simulink model "forward_facing_model"  (R2024b)
settings: Solver=VariableStepAuto  StartTime=0.0  StopTime=2474  RelTol=1e-3
model workspace (MATLAB code in the model file):
  | x = linspace(0,230.4,100);
  | m = 280;
libraries: autolibshared x2
settings Model: Creator=asus  LastModifiedBy=asus

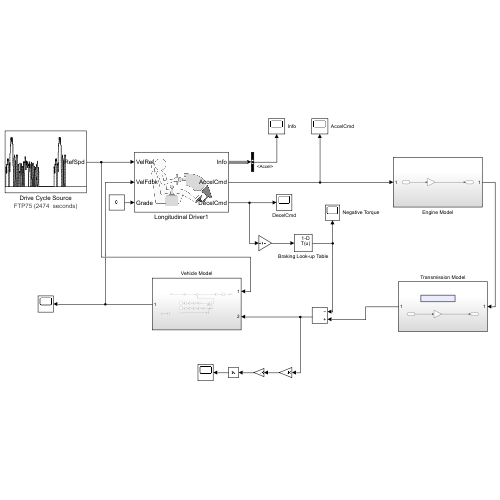
[thumbnail: Simulink's stored preview of the top-level diagram]
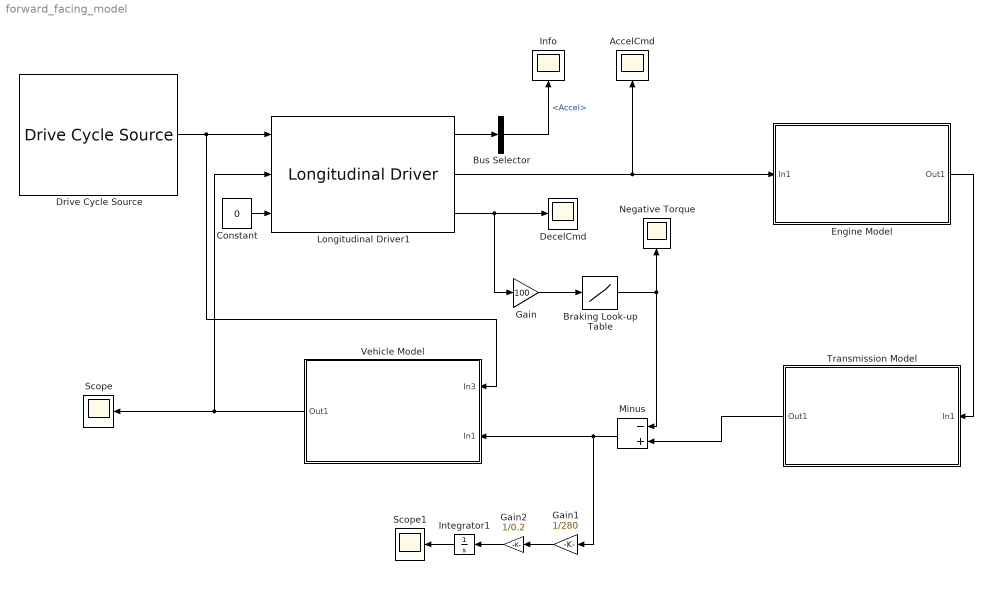
== system forward_facing_model ==
  AccelCmd : Scope
  Braking Look-up Table : Lookup_n-D  NumberOfTableDimensions=1  BreakpointsForDimension1=1:100  Table=x  InternalRulePriority=Speed  RndMeth=Simplest
  Bus Selector : BusSelector  OutputSignals=Accel
  Constant : Constant  Value=0
  DecelCmd : Scope
  Drive Cycle Source : autolibshared/Drive Cycle Source  cycleVar=FTP75  fileVar=cycleFTP75.mat  tfinal="2474  seconds"  cycleRepeat=off  outAccPort=off  outGearPort=off  gearList=No gear data  t_wot1=5  xdot_woto=0  xdot_wot1=30  t_wot2=20  xdot_wot2=0  t_wotend=30  srcUnit=m/s  outUnit=m/s  srcAccUnit=m/s/s  outAccUnit=m/s^2  dt=0  aMode=1  faultOption=off  velBnd=2  velBndUnit=mph  inUnit=m/s  timeBnd=1  failOption=off  stopSim=off  maxFaultCnt=10  maxFaultTime=2  maxTotFaultTime=15  traceOption=off  dtTrace=1  traceWindow=10  lastDCname=FTP75  lastOutUnit=mph  lastDT=0  lastTB=1  lastSB=2  forceCalcBound=off
  Engine Model : Subsystem
  Gain : Gain  Gain=100
  Gain1 : Gain  Gain=1/280
  Gain2 : Gain  Gain=1/0.2
  Info : Scope
  Integrator1 : Integrator
  Longitudinal Driver1 : autolibshared/Longitudinal Driver  extAccelOvr=off  extDecelOvr=off  extAccelHld=off  extDecelHld=off  extAccelZero=off  extDecelZero=off  cntrlType=PI  shftType=None  velUnits=m/s  gearOut=off  Kp=10  Ki=5  Kff=.1  Kg=0  VehVelVec=[0 100]  KffVec=[.1 .1]  KpVec=[10 10]  KiVec=[5 5]  KgVec=[0 0]  m=1500  Kpt=3000  tau=.1  L=2  aR=200  bR=2.5  cR=.5  g=9.81  vnom=5  Kaw=1  tauerr=.01  tauPt=2  GearInit=0  tShift=.1  pdlVec=[0.1 0.4 0.5 0.9]  upShftTbl=[-1 12.9375 26.4375 39.9375 51.18749999999999 62.4375 72.84375 83.25;-1 16.3125 29.8125 43.3125 54.5624 65.8125 76.78125 87.75;-1 19.6875 33.1875 46.68749999999999 57.9375 69.1875 80.71875 92.25;-1 33 52.5 77.25 100.5 138.75 161.875 185]  dwnShftTbl=[1 9.5625 23.0625 36.5625 47.8125 59.0625 68.90625 78.75;1 12.9375 26.4375 39.9375 51.18749999999999 62.4375 72.84375 83.25;1 16.3125 29.8125 43.3125 54.562499 65.8125 76.78125 87.75;1 19.6875 33.1875 46.68749999999999 57.9375 69.1875 80.71875 92.25]  tClutch=.5  tRev=.5  tPark=120  aMode=2  UpGearVec="[0  1  2  3  4  5  6  7]"  DownGearVec="[1  2  3  4  5  6  7  8]"
      settings: LibrarySourceBlock=vehdynlibdriver/Longitudinal Driver
  Minus : Sum  Inputs=-+
  Negative Torque : Scope
  Scope : Scope
  Scope1 : Scope
  Transmission Model : Subsystem
  Vehicle Model : Subsystem
  wires:
  Drive Cycle Source/1 -> Vehicle Model/1(In3), Longitudinal Driver1/1
  Longitudinal Driver1/1 -> Bus Selector/1
  Constant/1 -> Longitudinal Driver1/3
  Bus Selector/1 -> Info/1  "<Accel>"
  Longitudinal Driver1/2 -> Engine Model/1(In1), AccelCmd/1
  Longitudinal Driver1/3 -> DecelCmd/1, Gain/1
  Braking Look-up Table/1 -> Minus/1, Negative Torque/1
  Gain/1 -> Braking Look-up Table/1
  Engine Model/1(Out1) -> Transmission Model/1(In1)
  Transmission Model/1(Out1) -> Minus/2
  Minus/1 -> Gain1/1, Vehicle Model/2(In1)
  Vehicle Model/1(Out1) -> Scope/1, Longitudinal Driver1/2
  Integrator1/1 -> Scope1/1
  Gain2/1 -> Integrator1/1
  Gain1/1 -> Gain2/1

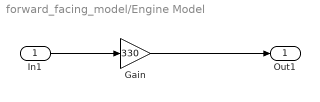
== system forward_facing_model/Engine Model ==
  In1 : Inport
  Gain : Gain  Gain=330
  Out1 : Outport
  wires:
  In1/1 -> Gain/1
  Gain/1 -> Out1/1

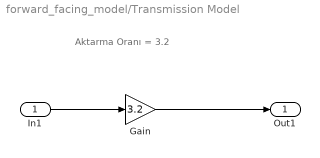
== system forward_facing_model/Transmission Model ==
  note: Aktarma Oranı = 3.2
  In1 : Inport
  Gain : Gain  Gain=3.2
  Out1 : Outport
  wires:
  In1/1 -> Gain/1
  Gain/1 -> Out1/1

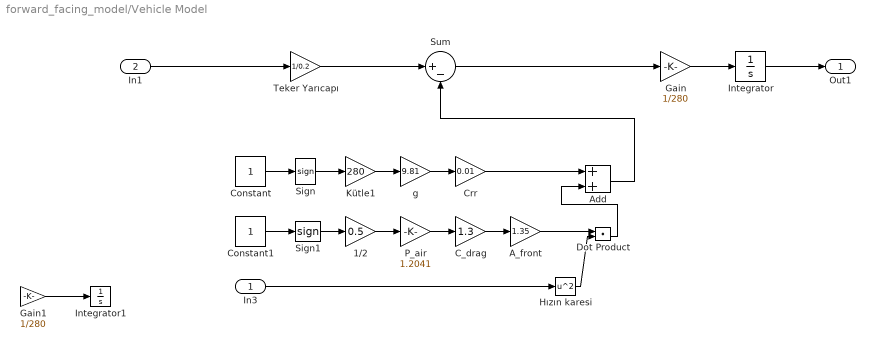
== system forward_facing_model/Vehicle Model ==
  In3 : Inport
  In1 : Inport  Port=2
  1/2 : Gain  Gain=0.5
  A_front : Gain  Gain=1.35
  Add : Sum
  C_drag : Gain  Gain=1.3
  Constant : Constant
  Constant1 : Constant
  Crr : Gain  Gain=0.01
  Dot Product : DotProduct  OutDataTypeStr=Inherit: Inherit via internal rule
  Gain : Gain  Gain=1/280
  Gain1 : Gain  Gain=1/280
  Hızın karesi : Math  Operator=square
  Integrator : Integrator
  Integrator1 : Integrator
  Kütle1 : Gain  Gain=280
  P_air : Gain  Gain=1.2041
  Sign : Signum
  Sign1 : Signum
  Sum : Sum  Inputs=|+-
  Teker Yarıcapı : Gain  Gain=1/0.2
  g : Gain  Gain=9.81
  Out1 : Outport
  wires:
  g/1 -> Crr/1
  Dot Product/1 -> Add/2
  A_front/1 -> Dot Product/1
  Crr/1 -> Add/1
  1/2/1 -> P_air/1
  C_drag/1 -> A_front/1
  Kütle1/1 -> g/1
  P_air/1 -> C_drag/1
  Hızın karesi/1 -> Dot Product/2
  In1/1 -> Teker Yarıcapı/1
  Gain/1 -> Integrator/1
  Integrator/1 -> Out1/1
  Teker Yarıcapı/1 -> Sum/1
  Sum/1 -> Gain/1
  Gain1/1 -> Integrator1/1
  Add/1 -> Sum/2
  In3/1 -> Hızın karesi/1
  Constant/1 -> Sign/1
  Constant1/1 -> Sign1/1
  Sign/1 -> Kütle1/1
  Sign1/1 -> 1/2/1
